simulink model "ctrlauto_tp1_d"  (R2019b)
settings: Solver=VariableStepAuto  StartTime=0.0  StopTime=2  RelTol=1e-3
undefined symbols (not defined in the file or in its folder): A, B, ueq, xeq
settings Model: Creator=rochi  LastModifiedBy=rochi

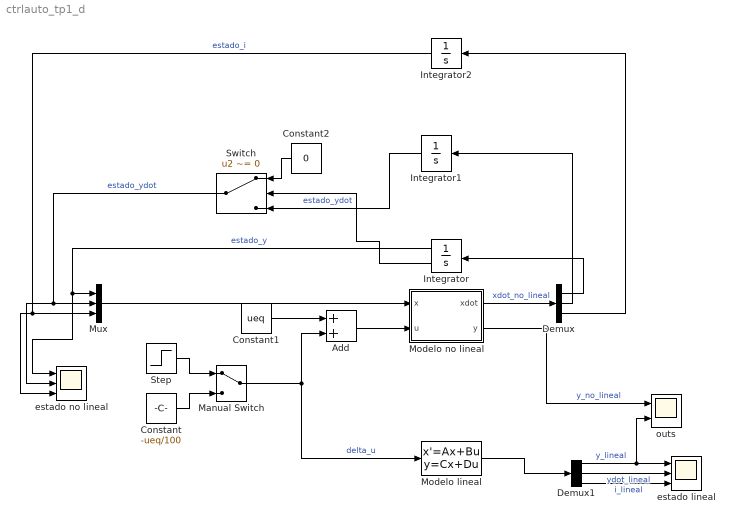
== system ctrlauto_tp1_d ==
  Add : Sum
  Constant : Constant  Value=-ueq/100  VectorParams1D=off
  Constant1 : Constant  Value=ueq  VectorParams1D=off
  Constant2 : Constant  Value=0
  Demux : Demux  Outputs=3
  Demux1 : Demux  Outputs=3
  Integrator : Integrator  LimitOutput=on  UpperSaturationLimit=.95  LowerSaturationLimit=-0.95  ShowSaturationPort=on
  Integrator1 : Integrator  LimitOutput=on  UpperSaturationLimit=1e5  LowerSaturationLimit=-1e5
  Integrator2 : Integrator  InitialCondition=xeq(3)  LimitOutput=on  UpperSaturationLimit=50  LowerSaturationLimit=-50
  Manual Switch : ManualSwitch
  Modelo lineal : StateSpace  A=A  B=B  C=eye(3)  D=zeros(3,1)  InitialCondition=zeros(1,3)  ContinuousStateAttributes={'y', 'ydot', 'i'}
  Modelo no lineal : MATLAB Function  TreatAsAtomicUnit=on
  Mux : Mux  Inputs=3
  Step : Step  Time=0.5  After=ueq/50  SampleTime=0
  Switch : Switch  Criteria=u2 ~= 0
  "estado lineal " : Scope  NumInputPorts=3
  estado no lineal : Scope  NumInputPorts=3
  outs : Scope  NumInputPorts=2
  wires:
  Modelo no lineal/2(y) -> outs/1  "y_no_lineal"
  Modelo no lineal/1(xdot) -> Demux/1  "xdot_no_lineal"
  Demux/1 -> Integrator/1
  Demux/2 -> Integrator1/1
  Demux/3 -> Integrator2/1
  Mux/1 -> Modelo no lineal/1(x)
  Integrator2/1 -> estado no lineal/3, Mux/3  "estado_i"
  Step/1 -> Manual Switch/1
  Constant/1 -> Manual Switch/2
  Integrator/1 -> estado no lineal/1, Mux/1  "estado_y"
  Modelo lineal/1 -> Demux1/1
  Demux1/2 -> "estado lineal "/2  "ydot_lineal"
  Demux1/1 -> outs/2, "estado lineal "/1  "y_lineal"
  Demux1/3 -> "estado lineal "/3  "i_lineal"
  Switch/1 -> estado no lineal/2, Mux/2  "estado_ydot"
  Integrator/2 -> Switch/2
  Integrator1/1 -> Switch/3  "estado_ydot"
  Constant2/1 -> Switch/1
  Manual Switch/1 -> Add/2, Modelo lineal/1  "delta_u"
  Add/1 -> Modelo no lineal/2(u)
  Constant1/1 -> Add/1

== matlab function ctrlauto_tp1_d/Modelo no lineal ==
  data: x input; xdot output; u input; y output
function [xdot,y] = nolineal(x, u)
    xdot1 = x(2);
    xdot2 = (5*(x(3) + 2)^2)/(2*(x(1) - 1)^2) - (5*(x(3)  - 2)^2)/(2*(x(1) + 1)^2) - 10; 
    xdot3 = - 4*x(3)^2 + u;

    xdot = [xdot1; xdot2; xdot3];
    y = x(1);
end
